simulink model "Simulation2_1"  (R2017b)
settings: Solver=VariableStepAuto  StartTime=0.0  StopTime=40  RelTol=1e-3  EnableMultiTasking=on
values from neighbouring files (symbols this model uses):
  A_Lin = 5    [PlotDopaEffect.m]    (also in PlotTwoChannels.m; Simulation1 Variables.mat = 20)
  CHNoise = 1e-4    (= 0.0001)    [PlotDopaEffect.m]    (also in PlotTwoChannels.m; Simulation1 Variables.mat = 1e-05)
  DAmp = 1    [PlotDopaEffect.m]    (also in PlotTwoChannels.m = 0.5; Simulation1 Variables.mat)
  epsilon = 0.2    [Simulation1 Variables.mat]
  epsilon_e = -0.2    [Simulation1 Variables.mat]
  epsilon_g = -0.2    [Simulation1 Variables.mat]
  epsilon_prime = -0.25    [Simulation1 Variables.mat]
  G_Lin = 5    [PlotDopaEffect.m]    (also in PlotTwoChannels.m; Simulation1 Variables.mat = 400)
  w_e = 1    [PlotDopaEffect.m]    (also in PlotTwoChannels.m; Simulation1 Variables.mat = 0.8)
  w_inh = 0.10    (= 0.1)    [PlotDopaEffect.m]    (also in PlotTwoChannels.m; Simulation1 Variables.mat = 0.03)
  w_minus = 1.05    [PlotDopaEffect.m]    (also in PlotTwoChannels.m; Simulation1 Variables.mat = 1)
  w_plus = 1    [PlotDopaEffect.m]    (also in PlotTwoChannels.m; Simulation1 Variables.mat = 0.8)
  w_s = 1    [PlotDopaEffect.m]    (also in PlotTwoChannels.m; Simulation1 Variables.mat)
  w_t = 1    [PlotDopaEffect.m]    (also in PlotTwoChannels.m; Simulation1 Variables.mat)
undefined symbols (not defined in the file or in its folder): sigbuilder_block
libraries: simulink x8
settings Model: Creator=acaso  LastModifiedBy=acaso
settings DataIOCC: LimitDataPoints=on
settings OptimizationCC: LifeSpan=inf
settings DebuggingCC: AllowSymbolicDim=off  SFUnexpectedBacktrackingDiag=warning  SFNoUnconditionalDefaultTransitionDiag=warning  SFExecutionAtInitializationDiag=none
settings ModelReferenceCC: PropagateSignalLabelsOutOfModel=off
settings CodeAppCC: StateflowObjectComments=on
settings GRTTargetCC: TargetLangStandard=C89/C90 (ANSI)
settings ConfigComp: CovMetricSettings=dw  CovHtmlReporting=on  CovSaveCumulativeToWorkspaceVar=on  CovSaveSingleToWorkspaceVar=on  CovExternalEMLEnable=off

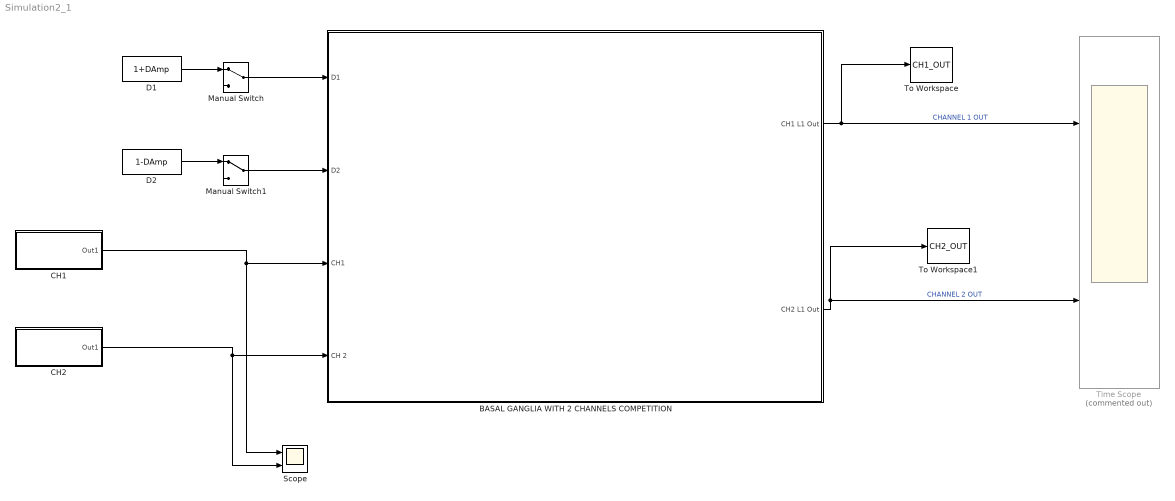
== system Simulation2_1 ==
  BASAL GANGLIA WITH 2 CHANNELS COMPETITION : Subsystem
  "CH1 " : Subsystem
  CH2 : Subsystem
  D1 : Constant  Value=1+DAmp  SampleTime=0.1
  D2 : Constant  Value=1-DAmp  SampleTime=0.1
  Manual Switch : ManualSwitch
  Manual Switch1 : ManualSwitch
  Scope : Scope  NumInputPorts=2
  Time Scope : Scope  Commented=on  NumInputPorts=2
  To Workspace : ToWorkspace  VariableName=CH1_OUT  SaveFormat=Timeseries  SampleTime=0.1
      settings: Save2DSignal=2-D array (concatenate along first dimension)
  To Workspace1 : ToWorkspace  VariableName=CH2_OUT  SaveFormat=Timeseries  SampleTime=0.1
      settings: Save2DSignal=2-D array (concatenate along first dimension)
  wires:
  BASAL GANGLIA WITH 2 CHANNELS COMPETITION/1(CH1 L1 Out) -> Time Scope/1, To Workspace/1  "CHANNEL 1 OUT"
  BASAL GANGLIA WITH 2 CHANNELS COMPETITION/2(CH2 L1 Out) -> To Workspace1/1, Time Scope/2  "CHANNEL 2 OUT"
  "CH1 "/1(Out1) -> Scope/1, BASAL GANGLIA WITH 2 CHANNELS COMPETITION/3("CH1 ")
  CH2/1(Out1) -> Scope/2, BASAL GANGLIA WITH 2 CHANNELS COMPETITION/4(CH 2)
  Manual Switch/1 -> BASAL GANGLIA WITH 2 CHANNELS COMPETITION/1(D1)
  D1/1 -> Manual Switch/1
  D2/1 -> Manual Switch1/1
  Manual Switch1/1 -> BASAL GANGLIA WITH 2 CHANNELS COMPETITION/2(D2)

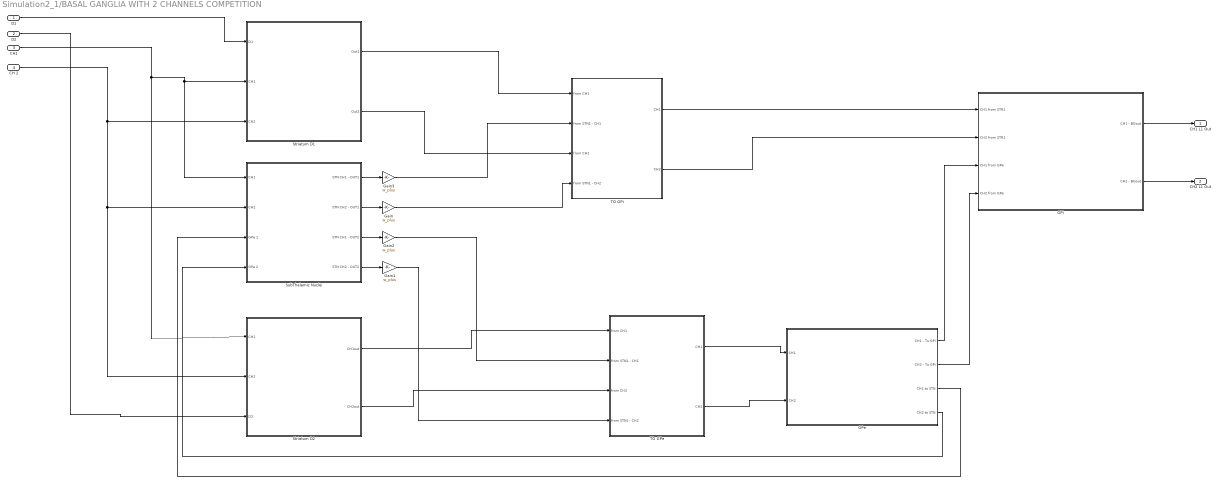
== system Simulation2_1/BASAL GANGLIA WITH 2 CHANNELS COMPETITION ==
  D1 : Inport
  D2 : Inport  Port=2
  "CH1 " : Inport  Port=3
  CH 2 : Inport  Port=4
  GPe : Subsystem  TreatAsAtomicUnit=on
  GPi : Subsystem
  Gain{,1..3} (4 alike) : Gain  Gain=w_plus
  "Striatum D1 " : Subsystem
  Striatum D2 : Subsystem
  SubThalamic Nuclei : Subsystem
  TO GPe : Subsystem
  TO GPi : Subsystem
  CH1 L1 Out : Outport
  CH2 L1 Out : Outport  Port=2
  wires:
  "Striatum D1 "/1(Out1) -> TO GPi/1(from CH1)
  Striatum D2/1(CH1out) -> TO GPe/1(from CH1)
  Striatum D2/2(CH2out) -> TO GPe/3(from CH2)
  SubThalamic Nuclei/3(STN CH1 - OUT2) -> Gain2/1
  SubThalamic Nuclei/4(STN CH2 - OUT2) -> Gain1/1
  SubThalamic Nuclei/1(STN CH1 - OUT1) -> Gain3/1
  SubThalamic Nuclei/2(STN CH2 - OUT1) -> Gain/1
  "Striatum D1 "/2(Out2) -> TO GPi/3(from CH2)
  TO GPi/1(CH1) -> GPi/1(CH1 from STR1)
  TO GPi/2(CH2) -> GPi/2(CH2 from STR1)
  TO GPe/1(CH1) -> GPe/1(CH1)
  TO GPe/2(CH2) -> GPe/2(CH2)
  GPe/1(CH1 - To GPi) -> GPi/3(CH1 from GPe)
  GPe/2("CH2 - To GPi ") -> GPi/4(CH2 from GPe)
  GPe/3(CH1 to STN) -> SubThalamic Nuclei/3(GPe 1)
  GPe/4(CH2 to STN) -> SubThalamic Nuclei/4(GPe 2)
  D1/1 -> "Striatum D1 "/1(D1)
  D2/1 -> Striatum D2/3(D2)
  "CH1 "/1 -> Striatum D2/1(CH1), "Striatum D1 "/2(CH1), SubThalamic Nuclei/1(CH1)
  CH 2/1 -> "Striatum D1 "/3(CH2), Striatum D2/2(CH2), SubThalamic Nuclei/2(CH2)
  GPi/2(CH2 - BGout) -> CH2 L1 Out/1
  GPi/1(CH1 - BGout) -> CH1 L1 Out/1
  Gain3/1 -> TO GPi/2(from STN1 - CH1)
  Gain/1 -> TO GPi/4(from STN1 - CH2)
  Gain2/1 -> TO GPe/2(from STN1 - CH1)
  Gain1/1 -> TO GPe/4(from STN1 - CH2)

== system Simulation2_1/CH1  ==
  Add : Sum
  Band-Limited White Noise : simulink/Sources/Band-Limited White Noise  Cov=[CHNoise]  Ts=0.1  seed=[23341]
  "CHANNEL1 IN " : Subsystem  Tag=STV Subsys  LoadFcn=sigbuilder_block('load');  StartFcn=sigbuilder_block('start');  StopFcn=sigbuilder_block('stop');  ClipboardFcn=sigbuilder_block('clipboard');  mask(Sigbuilder block){tuvar=[0:10]}
      mask help: Simulink:masks:SigbuilderBlock_MD
      mask init:
      | if ~strcmp(get_param(bdroot(gcbh),'SimulationStatus'),'stopped') tuvar = sigbuilder_block('maskInit'); end
      settings: CopyFcn=sigbuilder_block('copy');  DeleteFcn=sigbuilder_block('delete');  ModelCloseFcn=sigbuilder_block('modelClose');  PreSaveFcn=sigbuilder_block('preSave');  PauseFcn=sigbuilder_block('pause');  ContinueFcn=sigbuilder_block('continue');  NameChangeFcn=sigbuilder_block('namechange');  OpenFcn=sigbuilder_block('open',[306 237 1240 689 ]);  CloseFcn=sigbuilder_block('close');
      mask Display: plot(0, 0, 100, 100,[2, 2, 32, 32, 2], [68, 8, 8, 68, 68],[32, 2], [38, 38], [32, 19, 2],[53, 60, 44], [32, 17, 17, 2],[16, 16, 31, 31]);txt = getActiveGroup(gcbh);text(2, 100, txt,'verticalAlignment', 'top');
  To Workspace : ToWorkspace  VariableName=CH1_IN  SaveFormat=Timeseries  SampleTime=0.1
  Out1 : Outport
  wires:
  Band-Limited White Noise/1 -> Add/2
  Add/1 -> To Workspace/1, Out1/1
  "CHANNEL1 IN "/1(Signal 1) -> Add/1

== system Simulation2_1/CH2 ==
  Add : Sum
  Band-Limited White Noise : simulink/Sources/Band-Limited White Noise  Cov=[CHNoise]  Ts=0.1  seed=[23341]
  "CHANNEL2 IN " : Subsystem  Tag=STV Subsys  LoadFcn=sigbuilder_block('load');  StartFcn=sigbuilder_block('start');  StopFcn=sigbuilder_block('stop');  ClipboardFcn=sigbuilder_block('clipboard');  mask(Sigbuilder block){tuvar=[0:10]}
      mask help: Simulink:masks:SigbuilderBlock_MD
      mask init:
      | if ~strcmp(get_param(bdroot(gcbh),'SimulationStatus'),'stopped') tuvar = sigbuilder_block('maskInit'); end
      settings: CopyFcn=sigbuilder_block('copy');  DeleteFcn=sigbuilder_block('delete');  ModelCloseFcn=sigbuilder_block('modelClose');  PreSaveFcn=sigbuilder_block('preSave');  PauseFcn=sigbuilder_block('pause');  ContinueFcn=sigbuilder_block('continue');  NameChangeFcn=sigbuilder_block('namechange');  OpenFcn=sigbuilder_block('open',[268.8 5.4 877.8 580.8 ]);  CloseFcn=sigbuilder_block('close');
      mask Display: plot(0, 0, 100, 100,[2, 2, 32, 32, 2], [68, 8, 8, 68, 68],[32, 2], [38, 38], [32, 19, 2],[53, 60, 44], [32, 17, 17, 2],[16, 16, 31, 31]);txt = getActiveGroup(gcbh);text(2, 100, txt,'verticalAlignment', 'top');
  To Workspace : ToWorkspace  VariableName=CH2_IN  SaveFormat=Timeseries  SampleTime=0.1
  Out1 : Outport
  wires:
  Band-Limited White Noise/1 -> Add/2
  Add/1 -> To Workspace/1, Out1/1
  "CHANNEL2 IN "/1(Signal 1) -> Add/1

== system Simulation2_1/BASAL GANGLIA WITH 2 CHANNELS COMPETITION/GPe ==
  CH1 : Inport
  CH2 : Inport  Port=2
  GPe CH1 : Subsystem
  GPe CH2 : Subsystem
  CH1 - To GPi : Outport
  "CH2 - To GPi " : Outport  Port=2
  CH1 to STN : Outport  Port=3
  CH2 to STN : Outport  Port=4
  wires:
  CH1/1 -> GPe CH1/1(In)
  GPe CH1/1(To GPi) -> CH1 - To GPi/1
  CH2/1 -> GPe CH2/1(In)
  GPe CH2/1(To GPi) -> "CH2 - To GPi "/1
  GPe CH1/2(To STN) -> CH1 to STN/1
  GPe CH2/2(To STN) -> CH2 to STN/1

== system Simulation2_1/BASAL GANGLIA WITH 2 CHANNELS COMPETITION/GPi ==
  CH1 from STR1 : Inport
  CH2 from STR1 : Inport  Port=2
  CH1 from GPe : Inport  Port=3
  CH2 from GPe : Inport  Port=4
  GPi  CH1 : Subsystem
  GPi  CH2 : Subsystem
  CH1 - BGout : Outport
  CH2 - BGout : Outport  Port=2
  wires:
  CH1 from STR1/1 -> GPi  CH1/1(from StrD1)
  GPi  CH2/1(To Thal) -> CH2 - BGout/1
  GPi  CH1/1(To Thal) -> CH1 - BGout/1
  CH2 from STR1/1 -> GPi  CH2/1(from StrD1)
  CH1 from GPe/1 -> GPi  CH1/2(from GPe)
  CH2 from GPe/1 -> GPi  CH2/2(from GPe)

== system Simulation2_1/BASAL GANGLIA WITH 2 CHANNELS COMPETITION/Striatum D1  ==
  D1 : Inport
  CH1 : Inport  Port=2
  CH2 : Inport  Port=3
  Constant : Constant  Value=w_inh
  MATLAB Function : MATLAB Function  TreatAsAtomicUnit=on
  "Striatum D1 CH1 " : Subsystem
  Striatum D1 CH2 : Subsystem
  Out1 : Outport
  Out2 : Outport  Port=2
  wires:
  CH1/1 -> "Striatum D1 CH1 "/1(Channel)
  CH2/1 -> Striatum D1 CH2/1(Channel)
  D1/1 -> "Striatum D1 CH1 "/2(D1), Striatum D1 CH2/2(D1)
  "Striatum D1 CH1 "/1(Striatum D1 Out) -> MATLAB Function/1(ch1_in)
  Striatum D1 CH2/1(Striatum D1 Out) -> MATLAB Function/2(ch2_in)
  MATLAB Function/2(ch2_out) -> Out2/1
  MATLAB Function/1(ch1_out) -> Out1/1
  Constant/1 -> MATLAB Function/3(w_inhib)

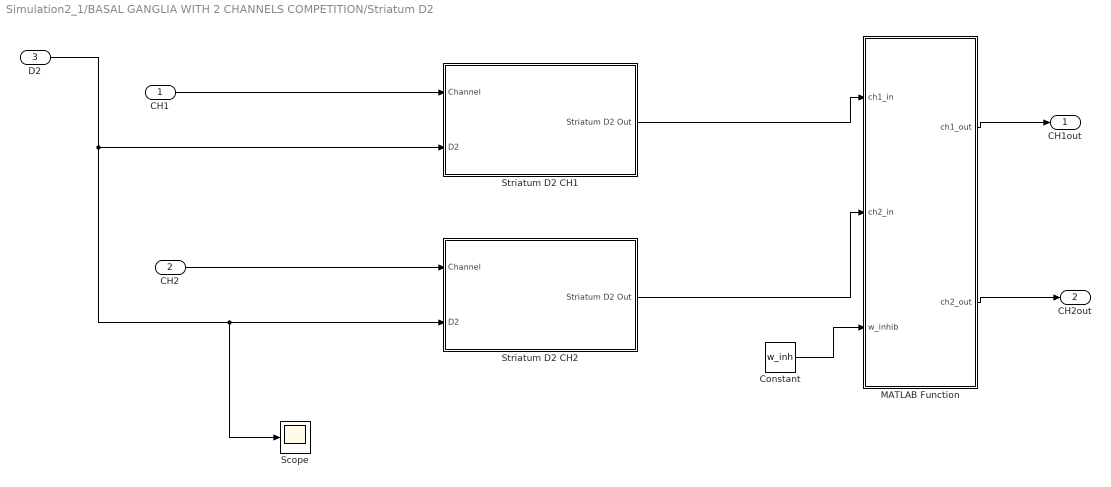
== system Simulation2_1/BASAL GANGLIA WITH 2 CHANNELS COMPETITION/Striatum D2 ==
  CH1 : Inport
  CH2 : Inport  Port=2
  D2 : Inport  Port=3
  Constant : Constant  Value=w_inh
  MATLAB Function : MATLAB Function  TreatAsAtomicUnit=on
  Scope : Scope
  Striatum D2 CH1 : Subsystem
  Striatum D2 CH2 : Subsystem
  CH1out : Outport
  CH2out : Outport  Port=2
  wires:
  Striatum D2 CH1/1(Striatum D2 Out) -> MATLAB Function/1(ch1_in)
  Striatum D2 CH2/1(Striatum D2 Out) -> MATLAB Function/2(ch2_in)
  MATLAB Function/1(ch1_out) -> CH1out/1
  MATLAB Function/2(ch2_out) -> CH2out/1
  CH1/1 -> Striatum D2 CH1/1(Channel)
  CH2/1 -> Striatum D2 CH2/1(Channel)
  D2/1 -> Scope/1, Striatum D2 CH2/2(D2), Striatum D2 CH1/2(D2)
  Constant/1 -> MATLAB Function/3(w_inhib)

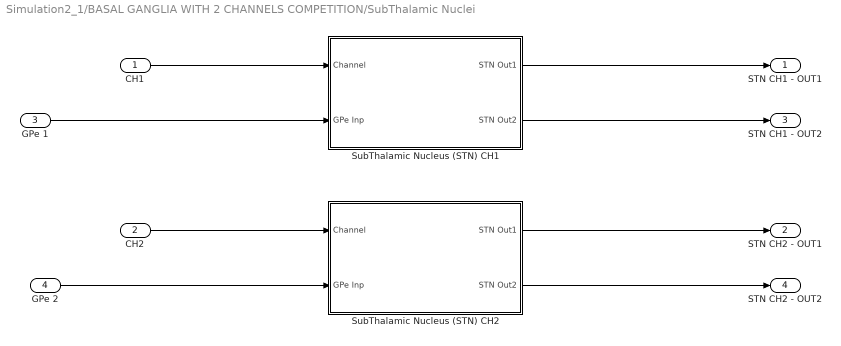
== system Simulation2_1/BASAL GANGLIA WITH 2 CHANNELS COMPETITION/SubThalamic Nuclei ==
  CH1 : Inport
  CH2 : Inport  Port=2
  GPe 1 : Inport  Port=3
  GPe 2 : Inport  Port=4
  SubThalamic Nucleus (STN) CH1 : Subsystem
  "SubThalamic Nucleus (STN) CH2 " : Subsystem
  STN CH1 - OUT1 : Outport
  STN CH2 - OUT1 : Outport  Port=2
  STN CH1 - OUT2 : Outport  Port=3
  STN CH2 - OUT2 : Outport  Port=4
  wires:
  CH1/1 -> SubThalamic Nucleus (STN) CH1/1(Channel)
  CH2/1 -> "SubThalamic Nucleus (STN) CH2 "/1(Channel)
  GPe 2/1 -> "SubThalamic Nucleus (STN) CH2 "/2(GPe Inp)
  GPe 1/1 -> SubThalamic Nucleus (STN) CH1/2(GPe Inp)
  SubThalamic Nucleus (STN) CH1/1(STN Out1) -> STN CH1 - OUT1/1
  "SubThalamic Nucleus (STN) CH2 "/1(STN Out1) -> STN CH2 - OUT1/1
  SubThalamic Nucleus (STN) CH1/2(STN Out2) -> STN CH1 - OUT2/1
  "SubThalamic Nucleus (STN) CH2 "/2(STN Out2) -> STN CH2 - OUT2/1

== system Simulation2_1/BASAL GANGLIA WITH 2 CHANNELS COMPETITION/TO GPe ==
  from CH1 : Inport
  from STN1 - CH1 : Inport  Port=2
  from CH2 : Inport  Port=3
  from STN1 - CH2 : Inport  Port=4
  Scope : Scope  NumInputPorts=2
  to GPi CH1 : Sum  Inputs=+++
  to GPi CH2 : Sum  Inputs=+++
  CH1 : Outport
  CH2 : Outport  Port=2
  wires:
  from STN1 - CH1/1 -> to GPi CH1/2, to GPi CH2/2
  from CH2/1 -> to GPi CH2/1
  from CH1/1 -> to GPi CH1/1
  from STN1 - CH2/1 -> to GPi CH2/3, to GPi CH1/3
  to GPi CH1/1 -> Scope/1, CH1/1
  to GPi CH2/1 -> Scope/2, CH2/1

== system Simulation2_1/BASAL GANGLIA WITH 2 CHANNELS COMPETITION/TO GPi ==
  from CH1 : Inport
  from STN1 - CH1 : Inport  Port=2
  from CH2 : Inport  Port=3
  from STN1 - CH2 : Inport  Port=4
  to GPi CH1 : Sum  Inputs=+++
  to GPi CH2 : Sum  Inputs=+++
  CH1 : Outport
  CH2 : Outport  Port=2
  wires:
  from STN1 - CH1/1 -> to GPi CH1/2, to GPi CH2/2
  from CH2/1 -> to GPi CH2/1
  from CH1/1 -> to GPi CH1/1
  from STN1 - CH2/1 -> to GPi CH2/3, to GPi CH1/3
  to GPi CH1/1 -> CH1/1
  to GPi CH2/1 -> CH2/1

== system Simulation2_1/CH1 /CHANNEL1 IN  ==
  Demux : Demux  Tag=STV Demux  Outputs=2
  FromWs : FromWorkspace  Tag=STV FromWs  VariableName=tuvar  SampleTime=0
      SigBuilderData=|
      | common.afterFinalStr = 'Extrapolate'
      | common.sampleTime = 0
      | dataSet.timeRange = [0 35]
      | dataSet.name = 'Group 1'
      | sbobj.Groups.Name = 'Group 1'
      | sbobj.Groups.Signals(1).Name = 'Signal 1'
      | sbobj.Groups.Signals(1).XData = [0 5 5 10 10 15 15 20 20 25 25 35]
      | sbobj.Groups.Signals(1).YData = [-0.002 -0.002 0.4 0.402 0.598 0.598 0.898 0.898 0.4 0.4 -0.002 -0.002]
      | sbobj.Groups.Signals(2).Name = 'Signal 2'
      | sbobj.Groups.Signals(2).XData = [0 5 5 20 20 35]
      | sbobj.Groups.Signals(2).YData = [0 0 1 1 0 0]
      | sbobj.Groups.TimeRange = [0 35]
  Signal 1 : Outport  Tag=STV Outport
  Signal 2 : Outport  Tag=STV Outport  Port=2
  wires:
  Demux/1 -> Signal 1/1
  FromWs/1 -> Demux/1
  Demux/2 -> Signal 2/1

== system Simulation2_1/CH2/CHANNEL2 IN  ==
  Demux : Demux  Tag=STV Demux  Outputs=2
  FromWs : FromWorkspace  Tag=STV FromWs  VariableName=tuvar  SampleTime=0
      SigBuilderData=|
      | common.afterFinalStr = 'Extrapolate'
      | common.sampleTime = 0
      | dataSet.timeRange = [0 35]
      | dataSet.name = 'Group 1'
      | sbobj.Groups.Name = 'Group 1'
      | sbobj.Groups.Signals(1).Name = 'Signal 1'
      | sbobj.Groups.Signals(1).XData = [0 10 10 15.05 15.05 20 20 24.95 24.95 30 30 35]
      | sbobj.Groups.Signals(1).YData = [-0.002 -0.002 0.40108 0.402 0.598 0.598 0.898 0.898 0.405 0.405 -0.002 -0.002]
      | sbobj.Groups.Signals(2).Name = 'Signal 2'
      | sbobj.Groups.Signals(2).XData = [0 0.4 0.4 34.55 34.55 35]
      | sbobj.Groups.Signals(2).YData = [0 0 0.615 0.605 0 0]
      | sbobj.Groups.TimeRange = [0 35]
  Signal 1 : Outport  Tag=STV Outport
  Signal 2 : Outport  Tag=STV Outport  Port=2
  wires:
  Demux/1 -> Signal 1/1
  FromWs/1 -> Demux/1
  Demux/2 -> Signal 2/1

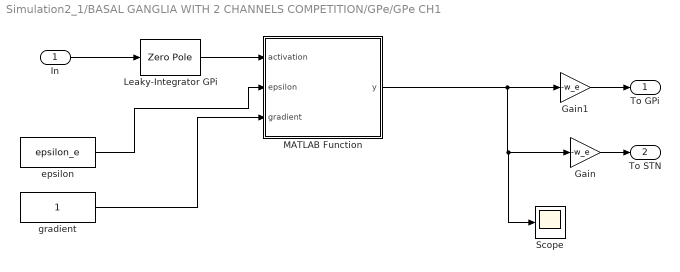
== system Simulation2_1/BASAL GANGLIA WITH 2 CHANNELS COMPETITION/GPe/GPe CH1 ==
  In : Inport
  Gain : Gain  Gain=-w_e
  Gain1 : Gain  Gain=-w_e
  Leaky-Integrator GPi : ZeroPole  Zeros=[]  Poles=[-A_Lin]  Gain=[G_Lin]
  MATLAB Function : MATLAB Function  TreatAsAtomicUnit=on
  Scope : Scope
  epsilon : Constant  Value=epsilon_e
  "gradient " : Constant
  To GPi : Outport
  To STN : Outport  Port=2
  wires:
  In/1 -> Leaky-Integrator GPi/1
  Leaky-Integrator GPi/1 -> MATLAB Function/1(activation)
  MATLAB Function/1(y) -> Scope/1, Gain/1, Gain1/1
  Gain1/1 -> To GPi/1
  Gain/1 -> To STN/1
  epsilon/1 -> MATLAB Function/2(epsilon)
  "gradient "/1 -> MATLAB Function/3(gradient)

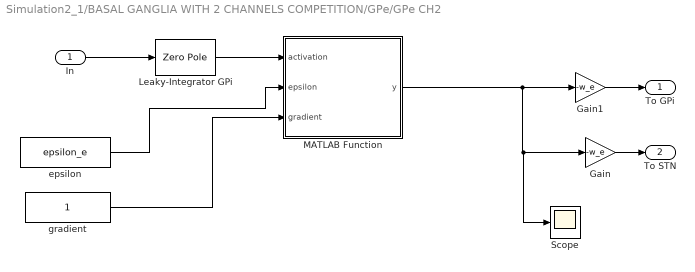
== system Simulation2_1/BASAL GANGLIA WITH 2 CHANNELS COMPETITION/GPe/GPe CH2 ==
  In : Inport
  Gain : Gain  Gain=-w_e
  Gain1 : Gain  Gain=-w_e
  Leaky-Integrator GPi : ZeroPole  Zeros=[]  Poles=[-A_Lin]  Gain=[G_Lin]
  MATLAB Function : MATLAB Function  TreatAsAtomicUnit=on
  Scope : Scope
  epsilon : Constant  Value=epsilon_e
  "gradient " : Constant
  To GPi : Outport
  To STN : Outport  Port=2
  wires:
  In/1 -> Leaky-Integrator GPi/1
  Leaky-Integrator GPi/1 -> MATLAB Function/1(activation)
  MATLAB Function/1(y) -> Scope/1, Gain/1, Gain1/1
  Gain1/1 -> To GPi/1
  Gain/1 -> To STN/1
  epsilon/1 -> MATLAB Function/2(epsilon)
  "gradient "/1 -> MATLAB Function/3(gradient)

== system Simulation2_1/BASAL GANGLIA WITH 2 CHANNELS COMPETITION/GPi/GPi  CH1 ==
  from StrD1 : Inport
  from GPe : Inport  Port=2
  Leaky-Integrator GPi : ZeroPole  Zeros=[]  Poles=[-A_Lin]  Gain=[G_Lin]
  MATLAB Function : MATLAB Function  TreatAsAtomicUnit=on
  Sum : Sum
  epsilon : Constant  Value=epsilon_g
  "gradient " : Constant
  To Thal : Outport
  wires:
  from StrD1/1 -> Sum/1
  Leaky-Integrator GPi/1 -> MATLAB Function/1(activation)
  MATLAB Function/1(y) -> To Thal/1
  epsilon/1 -> MATLAB Function/2(epsilon)
  "gradient "/1 -> MATLAB Function/3(gradient)
  from GPe/1 -> Sum/2
  Sum/1 -> Leaky-Integrator GPi/1

== system Simulation2_1/BASAL GANGLIA WITH 2 CHANNELS COMPETITION/GPi/GPi  CH2 ==
  from StrD1 : Inport
  from GPe : Inport  Port=2
  Leaky-Integrator GPi : ZeroPole  Zeros=[]  Poles=[-A_Lin]  Gain=[G_Lin]
  MATLAB Function : MATLAB Function  TreatAsAtomicUnit=on
  Sum : Sum
  epsilon : Constant  Value=epsilon_g
  "gradient " : Constant
  To Thal : Outport
  wires:
  from StrD1/1 -> Sum/1
  Leaky-Integrator GPi/1 -> MATLAB Function/1(activation)
  MATLAB Function/1(y) -> To Thal/1
  epsilon/1 -> MATLAB Function/2(epsilon)
  "gradient "/1 -> MATLAB Function/3(gradient)
  from GPe/1 -> Sum/2
  Sum/1 -> Leaky-Integrator GPi/1

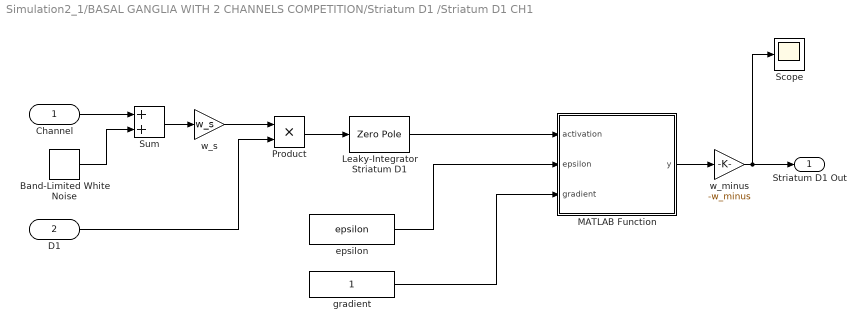
== system Simulation2_1/BASAL GANGLIA WITH 2 CHANNELS COMPETITION/Striatum D1 /Striatum D1 CH1  ==
  Channel : Inport
  D1 : Inport  Port=2
  Band-Limited White Noise : simulink/Sources/Band-Limited White Noise  Cov=[0]  Ts=0.1  seed=[23341]
  "Leaky-Integrator Striatum D1 " : ZeroPole  Zeros=[]  Poles=[-A_Lin]  Gain=[G_Lin]
  MATLAB Function : MATLAB Function  TreatAsAtomicUnit=on
  Product : Product
  Scope : Scope
  Sum : Sum
  epsilon : Constant  Value=epsilon
  "gradient " : Constant
  "w_minus " : Gain  Gain=-w_minus
  w_s : Gain  Gain=w_s
  Striatum D1 Out : Outport
  wires:
  MATLAB Function/1(y) -> "w_minus "/1
  "Leaky-Integrator Striatum D1 "/1 -> MATLAB Function/1(activation)
  Product/1 -> "Leaky-Integrator Striatum D1 "/1
  w_s/1 -> Product/1
  Channel/1 -> Sum/1
  Sum/1 -> w_s/1
  D1/1 -> Product/2
  "w_minus "/1 -> Scope/1, Striatum D1 Out/1
  epsilon/1 -> MATLAB Function/2(epsilon)
  "gradient "/1 -> MATLAB Function/3(gradient)
  Band-Limited White Noise/1 -> Sum/2

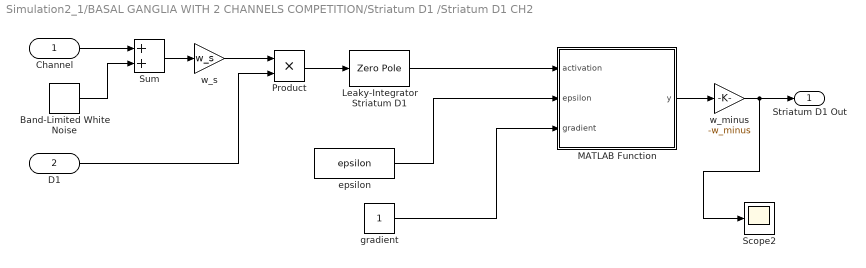
== system Simulation2_1/BASAL GANGLIA WITH 2 CHANNELS COMPETITION/Striatum D1 /Striatum D1 CH2 ==
  Channel : Inport
  D1 : Inport  Port=2
  Band-Limited White Noise : simulink/Sources/Band-Limited White Noise  Cov=[0]  Ts=0.1  seed=[23341]
  "Leaky-Integrator Striatum D1 " : ZeroPole  Zeros=[]  Poles=[-A_Lin]  Gain=[G_Lin]
  MATLAB Function : MATLAB Function  TreatAsAtomicUnit=on
  Product : Product
  Scope2 : Scope
  "Sum " : Sum
  epsilon : Constant  Value=epsilon
  "gradient " : Constant
  "w_minus " : Gain  Gain=-w_minus
  w_s : Gain  Gain=w_s
  Striatum D1 Out : Outport
  wires:
  MATLAB Function/1(y) -> "w_minus "/1
  "Leaky-Integrator Striatum D1 "/1 -> MATLAB Function/1(activation)
  Product/1 -> "Leaky-Integrator Striatum D1 "/1
  w_s/1 -> Product/1
  Channel/1 -> "Sum "/1
  Band-Limited White Noise/1 -> "Sum "/2
  "Sum "/1 -> w_s/1
  D1/1 -> Product/2
  "w_minus "/1 -> Scope2/1, Striatum D1 Out/1
  epsilon/1 -> MATLAB Function/2(epsilon)
  "gradient "/1 -> MATLAB Function/3(gradient)

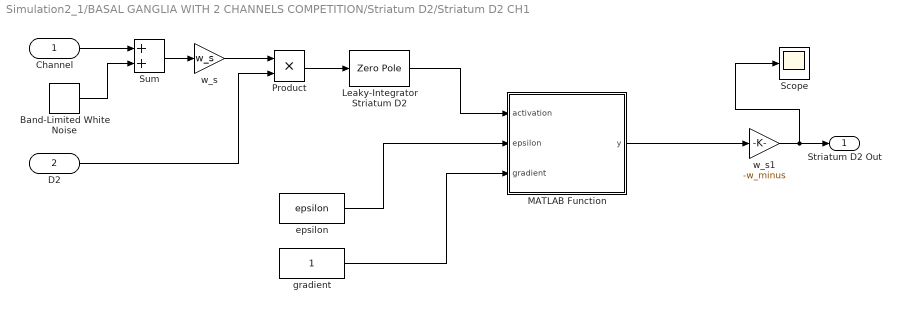
== system Simulation2_1/BASAL GANGLIA WITH 2 CHANNELS COMPETITION/Striatum D2/Striatum D2 CH1 ==
  Channel : Inport
  D2 : Inport  Port=2
  Band-Limited White Noise : simulink/Sources/Band-Limited White Noise  Cov=[0]  Ts=0.1  seed=[23341]
  Leaky-Integrator Striatum D2 : ZeroPole  Zeros=[]  Poles=[-A_Lin]  Gain=[G_Lin]
  MATLAB Function : MATLAB Function  TreatAsAtomicUnit=on
  Product : Product
  Scope : Scope
  "Sum " : Sum
  epsilon : Constant  Value=epsilon
  "gradient " : Constant
  w_s : Gain  Gain=w_s
  w_s1 : Gain  Gain=-w_minus
  Striatum D2 Out : Outport
  wires:
  MATLAB Function/1(y) -> w_s1/1
  Product/1 -> Leaky-Integrator Striatum D2/1
  w_s/1 -> Product/1
  Channel/1 -> "Sum "/1
  Band-Limited White Noise/1 -> "Sum "/2
  "Sum "/1 -> w_s/1
  D2/1 -> Product/2
  w_s1/1 -> Scope/1, Striatum D2 Out/1
  Leaky-Integrator Striatum D2/1 -> MATLAB Function/1(activation)
  epsilon/1 -> MATLAB Function/2(epsilon)
  "gradient "/1 -> MATLAB Function/3(gradient)

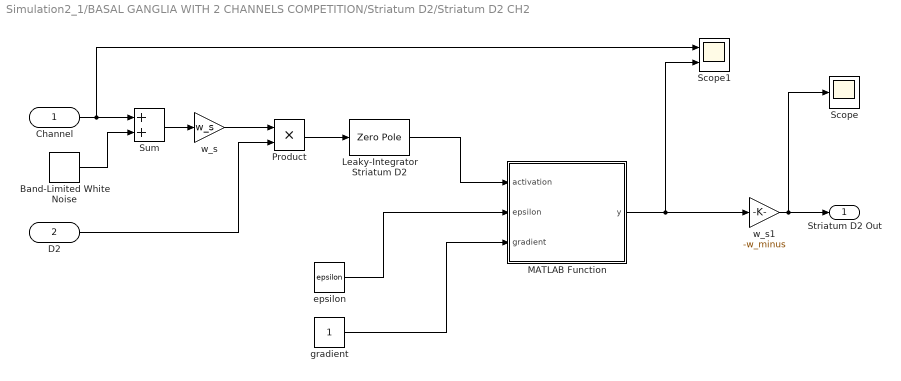
== system Simulation2_1/BASAL GANGLIA WITH 2 CHANNELS COMPETITION/Striatum D2/Striatum D2 CH2 ==
  Channel : Inport
  D2 : Inport  Port=2
  Band-Limited White Noise : simulink/Sources/Band-Limited White Noise  Cov=[0]  Ts=0.1  seed=[23341]
  Leaky-Integrator Striatum D2 : ZeroPole  Zeros=[]  Poles=[-A_Lin]  Gain=[G_Lin]
  MATLAB Function : MATLAB Function  TreatAsAtomicUnit=on
  Product : Product
  Scope : Scope
  Scope1 : Scope  NumInputPorts=2
  "Sum " : Sum
  epsilon : Constant  Value=epsilon
  "gradient " : Constant
  w_s : Gain  Gain=w_s
  w_s1 : Gain  Gain=-w_minus
  Striatum D2 Out : Outport
  wires:
  MATLAB Function/1(y) -> Scope1/2, w_s1/1
  Product/1 -> Leaky-Integrator Striatum D2/1
  w_s/1 -> Product/1
  Channel/1 -> Scope1/1, "Sum "/1
  Band-Limited White Noise/1 -> "Sum "/2
  "Sum "/1 -> w_s/1
  D2/1 -> Product/2
  w_s1/1 -> Scope/1, Striatum D2 Out/1
  Leaky-Integrator Striatum D2/1 -> MATLAB Function/1(activation)
  epsilon/1 -> MATLAB Function/2(epsilon)
  "gradient "/1 -> MATLAB Function/3(gradient)

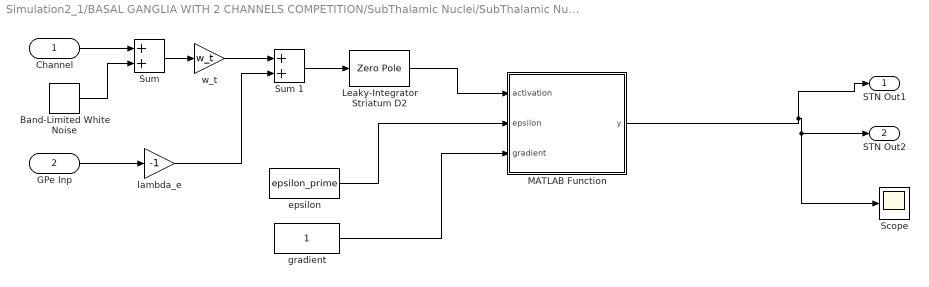
== system Simulation2_1/BASAL GANGLIA WITH 2 CHANNELS COMPETITION/SubThalamic Nuclei/SubThalamic Nucleus (STN) CH1 ==
  Channel : Inport
  GPe Inp : Inport  Port=2
  Band-Limited White Noise : simulink/Sources/Band-Limited White Noise  Cov=[0]  Ts=0.1  seed=[23341]
  Leaky-Integrator Striatum D2 : ZeroPole  Zeros=[]  Poles=[-A_Lin]  Gain=[G_Lin]
  MATLAB Function : MATLAB Function  TreatAsAtomicUnit=on
  Scope : Scope
  "Sum " : Sum
  Sum 1 : Sum
  epsilon : Constant  Value=epsilon_prime
  "gradient " : Constant
  lambda_e : Gain  Gain=-1
  w_t : Gain  Gain=w_t
  STN Out1 : Outport
  STN Out2 : Outport  Port=2
  wires:
  Leaky-Integrator Striatum D2/1 -> MATLAB Function/1(activation)
  Sum 1/1 -> Leaky-Integrator Striatum D2/1
  w_t/1 -> Sum 1/1
  Channel/1 -> "Sum "/1
  Band-Limited White Noise/1 -> "Sum "/2
  "Sum "/1 -> w_t/1
  GPe Inp/1 -> lambda_e/1
  lambda_e/1 -> Sum 1/2
  MATLAB Function/1(y) -> STN Out1/1, Scope/1, STN Out2/1
  epsilon/1 -> MATLAB Function/2(epsilon)
  "gradient "/1 -> MATLAB Function/3(gradient)

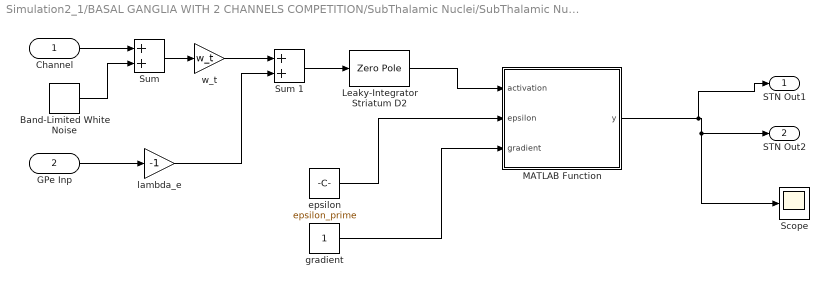
== system Simulation2_1/BASAL GANGLIA WITH 2 CHANNELS COMPETITION/SubThalamic Nuclei/SubThalamic Nucleus (STN) CH2  ==
  Channel : Inport
  GPe Inp : Inport  Port=2
  Band-Limited White Noise : simulink/Sources/Band-Limited White Noise  Cov=[0]  Ts=0.1  seed=[23341]
  Leaky-Integrator Striatum D2 : ZeroPole  Zeros=[]  Poles=[-A_Lin]  Gain=[G_Lin]
  MATLAB Function : MATLAB Function  TreatAsAtomicUnit=on
  Scope : Scope
  "Sum " : Sum
  Sum 1 : Sum
  epsilon : Constant  Value=epsilon_prime
  "gradient " : Constant
  lambda_e : Gain  Gain=-1
  w_t : Gain  Gain=w_t
  STN Out1 : Outport
  STN Out2 : Outport  Port=2
  wires:
  Leaky-Integrator Striatum D2/1 -> MATLAB Function/1(activation)
  Sum 1/1 -> Leaky-Integrator Striatum D2/1
  w_t/1 -> Sum 1/1
  Channel/1 -> "Sum "/1
  Band-Limited White Noise/1 -> "Sum "/2
  "Sum "/1 -> w_t/1
  GPe Inp/1 -> lambda_e/1
  lambda_e/1 -> Sum 1/2
  MATLAB Function/1(y) -> STN Out1/1, Scope/1, STN Out2/1
  epsilon/1 -> MATLAB Function/2(epsilon)
  "gradient "/1 -> MATLAB Function/3(gradient)

== matlab function Simulation2_1/BASAL GANGLIA WITH 2 CHANNELS COMPETITION/Striatum D1 /Striatum D1 CH2/MATLAB Function ==
  data: activation input; y output; epsilon input; gradient input
function y = thresh_eps(activation, epsilon, gradient)

y = gradient*(activation - epsilon);

%% Apply the slope function
if activation >= 1/gradient + epsilon 
    y = 1; 
elseif activation < epsilon 
    y = 0;
else
    y = gradient * (activation - epsilon);
end
end

== matlab function Simulation2_1/BASAL GANGLIA WITH 2 CHANNELS COMPETITION/Striatum D1 /Striatum D1 CH1 /MATLAB Function ==
  data: activation input; y output; epsilon input; gradient input
function y = thresh_eps(activation, epsilon, gradient)

%% Apply the slope function
if activation >= 1/gradient + epsilon 
    y = 1; 
elseif activation < epsilon 
    y = 0;
else
    y = gradient * (activation - epsilon);
end

end

== matlab function Simulation2_1/BASAL GANGLIA WITH 2 CHANNELS COMPETITION/Striatum D2/MATLAB Function ==
  data: ch1_in input; ch1_out output; ch2_in input; ch2_out output; w_inhib input
function [ch1_out, ch2_out] = recurrent_inh2(ch1_in, ch2_in, w_inhib)

ch1_out = ch1_in - w_inhib*(ch2_in);

ch2_out = ch2_in - w_inhib*(ch1_in);

end

== matlab function Simulation2_1/BASAL GANGLIA WITH 2 CHANNELS COMPETITION/Striatum D2/Striatum D2 CH1/MATLAB Function ==
  data: activation input; y output; epsilon input; gradient input
function y = thresh_eps(activation, epsilon, gradient)

%% Apply the slope function
if activation >= 1/gradient + epsilon 
    y = 1; 
elseif activation < epsilon 
    y = 0;
else
    y = gradient * (activation - epsilon);
end

end

== matlab function Simulation2_1/BASAL GANGLIA WITH 2 CHANNELS COMPETITION/Striatum D2/Striatum D2 CH2/MATLAB Function ==
  data: activation input; y output; epsilon input; gradient input
function y = thresh_eps(activation, epsilon, gradient)

%% Apply the slope function
if activation >= 1/gradient + epsilon 
    y = 1; 
elseif activation < epsilon 
    y = 0;
else
    y = gradient * (activation - epsilon);
end

end

== matlab function Simulation2_1/BASAL GANGLIA WITH 2 CHANNELS COMPETITION/SubThalamic Nuclei/SubThalamic Nucleus (STN) CH2 /MATLAB Function ==
  data: activation input; y output; epsilon input; gradient input
function y = thresh_eps(activation, epsilon, gradient)

%% Apply the slope function
if activation >= 1/gradient + epsilon 
    y = 1; 
elseif activation < epsilon 
    y = 0;
else
    y = gradient * (activation - epsilon);
end

end

== matlab function Simulation2_1/BASAL GANGLIA WITH 2 CHANNELS COMPETITION/SubThalamic Nuclei/SubThalamic Nucleus (STN) CH1/MATLAB Function ==
  data: activation input; y output; epsilon input; gradient input
function y = thresh_eps(activation, epsilon, gradient)

%% Apply the slope function

if activation >= 1/gradient + epsilon 
    y = 1; 
elseif activation < epsilon 
    y = 0;
else
    y = gradient * (activation - epsilon);
end

end

== matlab function Simulation2_1/BASAL GANGLIA WITH 2 CHANNELS COMPETITION/GPi/GPi  CH2/MATLAB Function ==
  data: activation input; y output; epsilon input; gradient input
function y = thresh_eps(activation, epsilon, gradient)

%% Apply the slope function
if activation >= 1/gradient + epsilon 
    y = 1; 
elseif activation < epsilon 
    y = 0;
else
    y = gradient * (activation - epsilon);
end

end

== matlab function Simulation2_1/BASAL GANGLIA WITH 2 CHANNELS COMPETITION/GPe/GPe CH2/MATLAB Function ==
  data: activation input; y output; epsilon input; gradient input
function y = thresh_eps(activation, epsilon, gradient)

%% Apply the slope function
if activation >= 1/gradient + epsilon 
    y = 1; 
elseif activation < epsilon 
    y = 0;
else
    y = gradient * (activation - epsilon);
end

end

== matlab function Simulation2_1/BASAL GANGLIA WITH 2 CHANNELS COMPETITION/GPi/GPi  CH1/MATLAB Function ==
  data: activation input; y output; epsilon input; gradient input
function y = thresh_eps(activation, epsilon, gradient)

%% Apply the slope function
if activation >= 1/gradient + epsilon 
    y = 1; 
elseif activation < epsilon 
    y = 0;
else
    y = gradient * (activation - epsilon);
end

end

== matlab function Simulation2_1/BASAL GANGLIA WITH 2 CHANNELS COMPETITION/GPe/GPe CH1/MATLAB Function ==
  data: activation input; y output; epsilon input; gradient input
function y = thresh_eps(activation, epsilon, gradient)

%% Apply the slope function
if activation >= 1/gradient + epsilon 
    y = 1; 
elseif activation < epsilon 
    y = 0;
else
    y = gradient * (activation - epsilon);
end

end

== matlab function Simulation2_1/BASAL GANGLIA WITH 2 CHANNELS COMPETITION/Striatum D1 /MATLAB Function ==
  data: ch1_in input; ch1_out output; ch2_in input; ch2_out output; w_inhib input
function [ch1_out, ch2_out] = recurrent_inh2(ch1_in, ch2_in, w_inhib)


ch1_out = ch1_in - w_inhib*(ch2_in);

ch2_out = ch2_in - w_inhib*(ch1_in);

end
